simulink model "SimpleStateMachine"  (R2016a)
settings: Solver=ode4  StartTime=0.0  StopTime=inf  FixedStep=0.0002  RelTol=1e-3
libraries: slrtlib x1
settings Model: Creator=march  LastModifiedBy=march
settings SolverCC: EnableConcurrentExecution=on
settings DataIOCC: SaveFormat=StructureWithTime
settings OptimizationCC: BlockReduction=off  OptimizeBlockIOStorage=off  BufferReuse=off  GlobalBufferReuse=off  ExpressionFolding=off  LocalBlockOutputs=off
settings HardwareCC: ProdBitPerPointer=32  ProdLargestAtomicFloat=None  ProdWordSize=32  ProdLongLongMode=on  ProdHWDeviceType=Generic->32-bit x86 compatible
settings RTWCC: SystemTargetFile=slrt.tlc  TemplateMakefile=slrt_default_tmf  Description=Simulink Real-Time  RTWCompilerOptimization=on

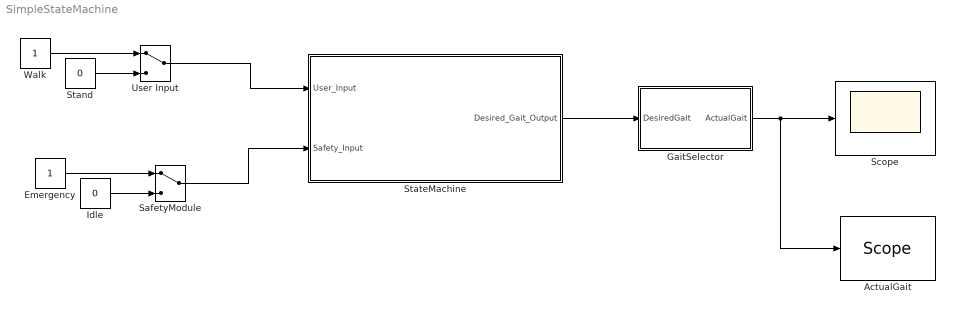
== system SimpleStateMachine ==
  "ActualGait " : slrtlib/Displays and Logging/Scope   scopeno=1  scopetype=Target  autostart=on  viewmode=Graphical redraw  formatstr='%15.6f'  grid=on  ylimits=[0,0]  nosamples=250  noprepostsamples=0  interleave=1  triggermode=FreeRun  triggersignal=1  trigsignalfromport=off  triggerlevel=0.0  triggerslope=Either  triggerscope=1  triggersample=0  filename=data.dat  mode=Lazy  writesize=512  autorestart=off  dynamicfilemode=off  maxwritefilesize=512*1024^2
  Emergency : Constant
  GaitSelector : Subsystem
  Idle : Constant  Value=0
  SafetyModule : ManualSwitch
  Scope : Scope
  Stand : Constant  Value=0
  StateMachine : Stateflow chart  TreatAsAtomicUnit=on
  User Input : ManualSwitch
  Walk : Constant
  wires:
  SafetyModule/1 -> StateMachine/2(Safety_Input)
  User Input/1 -> StateMachine/1(User_Input)
  Walk/1 -> User Input/1
  Stand/1 -> User Input/2
  Emergency/1 -> SafetyModule/1
  Idle/1 -> SafetyModule/2
  StateMachine/1(Desired_Gait_Output) -> GaitSelector/1(DesiredGait)
  GaitSelector/1(ActualGait) -> "ActualGait "/1, Scope/1

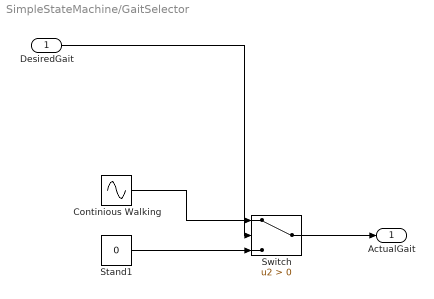
== system SimpleStateMachine/GaitSelector ==
  DesiredGait : Inport
  Continious Walking : Sin  SampleTime=0
  Stand1 : Constant  Value=0
  Switch : Switch  Criteria=u2 > Threshold
  ActualGait : Outport
  wires:
  DesiredGait/1 -> Switch/2
  Switch/1 -> ActualGait/1
  Stand1/1 -> Switch/3
  Continious Walking/1 -> Switch/1

== stateflow chart SimpleStateMachine/StateMachine ==
  state Standing
    entry: Desired_Gait_Output = 0
  state Walking
    entry: Desired_Gait_Output = 1
  (default) -> Standing
  Standing -> Standing [order 2]
  Walking -> Standing [order 1] : [User_Input==0 || Safety_Input==1]
  Standing -> Walking [order 1] : [User_Input>0 && Safety_Input==0]
  Walking -> Walking [order 2]
  data: User_Input input; Safety_Input input; Desired_Gait_Output output
